simulink model "qless_forgetting_factor_16x16_nofifo"  (R2021a)
settings: Solver=FixedStepDiscrete  StartTime=0.0  StopTime=stoptime*inf  RelTol=1e-3
InitFcn:
  | qless_init_16chan_fi
undefined symbols (not defined in the file): fc, numArrayElements, physconst, srcAngles, Ts
libraries: hdlsllib x137, commfilt2 x4, commrfcorlib x3, commsync2 x3, commrflib2 x2, commrandsrc3 x2, simulink x2, phasedtxrxlib x2, commdigbbndcpm2 x1, embreciprocals x1, commdigbbndpm3 x1
(part 5 of 22)

== system qless_forgetting_factor_16x16_nofifo/MVDR_QLess_HDL/Complex Partial-Systolic Matrix Solve Using Q-less QR Decomposition with Forgetting Factor Manually Tiled n=16/Complex Partial-Systolic Q-less QR with Forgetting Factor/Complex Partial-Systolic Q-less QR with Forgetting Factor Manually tiled/Complex Partial-Systolic Q-less QR Decomposition with Forgetting Factor Section Constant pivot11/Partial-Systolic Q-less QR with Forgetting Factor Memory Controller ==
  xIn : Inport
  aIn : Inport  Port=2
  validIn : Inport  Port=3
  validElim : Inport  Port=4
  restart : Inport  Port=5
  Delay{,2..4,6} (5 alike) : Delay  DelayLength=1
  MATLAB Function : MATLAB Function  TreatAsAtomicUnit=on
  xOut : Outport  VectorParamsAs1DForOutWhenUnconnected=off
  yOut : Outport  Port=2  VectorParamsAs1DForOutWhenUnconnected=off
  process : Outport  Port=3  VectorParamsAs1DForOutWhenUnconnected=off
  validOut : Outport  Port=4  VectorParamsAs1DForOutWhenUnconnected=off
  ready : Outport  Port=5  VectorParamsAs1DForOutWhenUnconnected=off
  wires:
  Delay/1 -> MATLAB Function/1(xIn)
  Delay2/1 -> MATLAB Function/2(aIn)
  Delay3/1 -> MATLAB Function/3(validIn)
  Delay4/1 -> MATLAB Function/4(validRowRotationInput)
  Delay6/1 -> MATLAB Function/5(restart)
  xIn/1 -> Delay/1  "A"
  aIn/1 -> Delay2/1
  validIn/1 -> Delay3/1  "validIn"
  validElim/1 -> Delay4/1  "validElim"
  restart/1 -> Delay6/1  "validElim"
  MATLAB Function/1(xOut) -> xOut/1
  MATLAB Function/2(yOut) -> yOut/1
  MATLAB Function/3(processRowRotations) -> process/1
  MATLAB Function/4(validOut) -> validOut/1
  MATLAB Function/5(ready) -> ready/1

== system qless_forgetting_factor_16x16_nofifo/MVDR_QLess_HDL/Complex Partial-Systolic Matrix Solve Using Q-less QR Decomposition with Forgetting Factor Manually Tiled n=16/Complex Partial-Systolic Q-less QR with Forgetting Factor/Complex Partial-Systolic Q-less QR with Forgetting Factor Manually tiled/Complex Partial-Systolic Q-less QR Decomposition with Forgetting Factor Section Constant pivot11/Same Datatype ==
  Data : Inport
  Reference : Inport  Port=2
  Data Type Duplicate : DataTypeDuplicate
  DataOut : Outport  VectorParamsAs1DForOutWhenUnconnected=off
  wires:
  Reference/1 -> Data Type Duplicate/2
  Data/1 -> DataOut/1, Data Type Duplicate/1

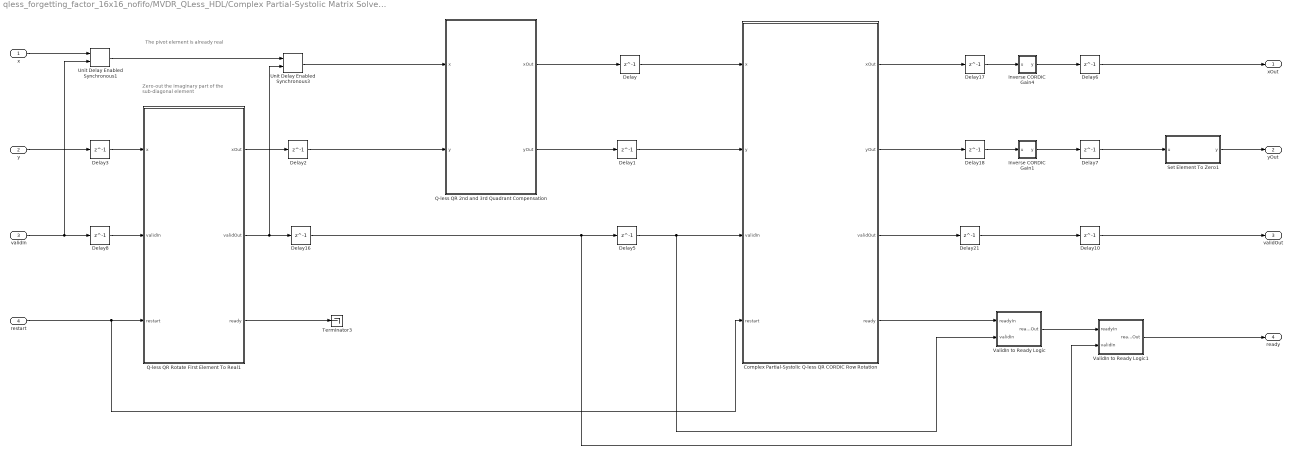
== system qless_forgetting_factor_16x16_nofifo/MVDR_QLess_HDL/Complex Partial-Systolic Matrix Solve Using Q-less QR Decomposition with Forgetting Factor Manually Tiled n=16/Complex Partial-Systolic Q-less QR with Forgetting Factor/Complex Partial-Systolic Q-less QR with Forgetting Factor Manually tiled/Complex Partial-Systolic Q-less QR Decomposition with Forgetting Factor Section Constant pivot12/Complex Partial-Systolic Q-less QR Row Rotations ==
  note: The pivot element is already real
  note: Zero-out the imaginary part
      | of the sub-diagonal element
  x : Inport
  y : Inport  Port=2
  validIn : Inport  Port=3
  restart : Inport  Port=4
  Complex Partial-Systolic Q-less QR CORDIC Row Rotation : Subsystem  TreatAsAtomicUnit=on  mask(Real Indexed CORDIC Row Rotation){n=n, pivot=pivot}
      mask prompts: n "fixed:emblib:ColumnsInA"
      mask help: fixed:emblib:RealIdxCORDIC
      mask DialogControl n Prompt: Number of columns in matrix A
  Delay{,1..3,5..8,10,16..18,21} (13 alike) : Delay  DelayLength=1
  Inverse CORDIC Gain1 : Subsystem  mask(Inverse CORDIC Gain){}
      mask help: fixed:emblib:InverseCORDICGainDescription
      mask Display: disp('1/An')
  Inverse CORDIC Gain4 : Subsystem  mask(Inverse CORDIC Gain){}
      mask help: fixed:emblib:InverseCORDICGainDescription
      mask Display: disp('1/An')
  Q-less QR 2nd and 3rd Quadrant Compensation : MATLAB Function  TreatAsAtomicUnit=on
  Q-less QR Rotate First Element To Real1 : Subsystem  TreatAsAtomicUnit=on  mask(Rotate First Element To Real){n=n, pivot=pivot}
      mask prompts: n "fixed:emblib:ColumnsInA"
      mask help: fixed:emblib:RotateFirstElementToRealDescription
      mask DialogControl n Prompt: Number of columns in matrix A
  Set Element To Zero1 : Subsystem  mask(Set Element To Zero){n=n, pivot=pivot}
      mask prompts: n "fixed:emblib:ColumnsInA"
      mask help: fixed:emblib:SetElementToZeroDescription
      mask DialogControl n Prompt: Number of columns in matrix A
  Terminator3 : Terminator
  Unit Delay Enabled Synchronous1 : hdlsllib/Discrete/Unit Delay Enabled Synchronous  InitialCondition=0.0  SampleTime=-1
      settings: SourceProductBaseCode=SL
  Unit Delay Enabled Synchronous3 : hdlsllib/Discrete/Unit Delay Enabled Synchronous  InitialCondition=0.0  SampleTime=-1
      settings: SourceProductBaseCode=SL
  ValidIn to Ready Logic : Subsystem
  ValidIn to Ready Logic1 : Subsystem
  xOut : Outport  VectorParamsAs1DForOutWhenUnconnected=off
  yOut : Outport  Port=2  VectorParamsAs1DForOutWhenUnconnected=off
  validOut : Outport  Port=3  VectorParamsAs1DForOutWhenUnconnected=off
  ready : Outport  Port=4  VectorParamsAs1DForOutWhenUnconnected=off
  wires:
  Delay6/1 -> xOut/1
  Complex Partial-Systolic Q-less QR CORDIC Row Rotation/1(xOut) -> Delay17/1
  Q-less QR 2nd and 3rd Quadrant Compensation/1(xOut) -> Delay/1
  Q-less QR 2nd and 3rd Quadrant Compensation/2(yOut) -> Delay1/1
  Delay/1 -> Complex Partial-Systolic Q-less QR CORDIC Row Rotation/1(x)
  Q-less QR Rotate First Element To Real1/2(validOut) -> Unit Delay Enabled Synchronous3/2, Delay16/1
  Q-less QR Rotate First Element To Real1/1(xOut) -> Delay2/1
  Delay1/1 -> Complex Partial-Systolic Q-less QR CORDIC Row Rotation/2(y)
  restart/1 -> Q-less QR Rotate First Element To Real1/3(restart), Complex Partial-Systolic Q-less QR CORDIC Row Rotation/4(restart)
  Delay5/1 -> ValidIn to Ready Logic/2(validIn), Complex Partial-Systolic Q-less QR CORDIC Row Rotation/3(validIn)
  Complex Partial-Systolic Q-less QR CORDIC Row Rotation/4(ready) -> ValidIn to Ready Logic/1(readyIn)
  Complex Partial-Systolic Q-less QR CORDIC Row Rotation/3(validOut) -> Delay21/1
  Complex Partial-Systolic Q-less QR CORDIC Row Rotation/2(yOut) -> Delay18/1
  y/1 -> Delay3/1
  Delay10/1 -> validOut/1
  ValidIn to Ready Logic/1(readyOut) -> ValidIn to Ready Logic1/1(readyIn)
  Delay7/1 -> Set Element To Zero1/1(u)
  Q-less QR Rotate First Element To Real1/3(ready) -> Terminator3/1
  ValidIn to Ready Logic1/1(readyOut) -> ready/1
  Delay21/1 -> Delay10/1
  Delay18/1 -> Inverse CORDIC Gain1/1(u)
  Delay17/1 -> Inverse CORDIC Gain4/1(u)
  Inverse CORDIC Gain4/1(y) -> Delay6/1
  Inverse CORDIC Gain1/1(y) -> Delay7/1
  validIn/1 -> Unit Delay Enabled Synchronous1/2, Delay8/1
  Delay16/1 -> ValidIn to Ready Logic1/2(validIn), Delay5/1
  Delay2/1 -> Q-less QR 2nd and 3rd Quadrant Compensation/2(y)
  Unit Delay Enabled Synchronous3/1 -> Q-less QR 2nd and 3rd Quadrant Compensation/1(x)
  Unit Delay Enabled Synchronous1/1 -> Unit Delay Enabled Synchronous3/1
  x/1 -> Unit Delay Enabled Synchronous1/1
  Delay3/1 -> Q-less QR Rotate First Element To Real1/1(x)
  Delay8/1 -> Q-less QR Rotate First Element To Real1/2(validIn)
  Set Element To Zero1/1(y) -> yOut/1

== system qless_forgetting_factor_16x16_nofifo/MVDR_QLess_HDL/Complex Partial-Systolic Matrix Solve Using Q-less QR Decomposition with Forgetting Factor Manually Tiled n=16/Complex Partial-Systolic Q-less QR with Forgetting Factor/Complex Partial-Systolic Q-less QR with Forgetting Factor Manually tiled/Complex Partial-Systolic Q-less QR Decomposition with Forgetting Factor Section Constant pivot12/Partial-Systolic Q-less QR with Forgetting Factor Memory Controller ==
  xIn : Inport
  aIn : Inport  Port=2
  validIn : Inport  Port=3
  validElim : Inport  Port=4
  restart : Inport  Port=5
  Delay{,2..4,6} (5 alike) : Delay  DelayLength=1
  MATLAB Function : MATLAB Function  TreatAsAtomicUnit=on
  xOut : Outport  VectorParamsAs1DForOutWhenUnconnected=off
  yOut : Outport  Port=2  VectorParamsAs1DForOutWhenUnconnected=off
  process : Outport  Port=3  VectorParamsAs1DForOutWhenUnconnected=off
  validOut : Outport  Port=4  VectorParamsAs1DForOutWhenUnconnected=off
  ready : Outport  Port=5  VectorParamsAs1DForOutWhenUnconnected=off
  wires:
  Delay/1 -> MATLAB Function/1(xIn)
  Delay2/1 -> MATLAB Function/2(aIn)
  Delay3/1 -> MATLAB Function/3(validIn)
  Delay4/1 -> MATLAB Function/4(validRowRotationInput)
  Delay6/1 -> MATLAB Function/5(restart)
  xIn/1 -> Delay/1  "A"
  aIn/1 -> Delay2/1
  validIn/1 -> Delay3/1  "validIn"
  validElim/1 -> Delay4/1  "validElim"
  restart/1 -> Delay6/1  "validElim"
  MATLAB Function/1(xOut) -> xOut/1
  MATLAB Function/2(yOut) -> yOut/1
  MATLAB Function/3(processRowRotations) -> process/1
  MATLAB Function/4(validOut) -> validOut/1
  MATLAB Function/5(ready) -> ready/1

== system qless_forgetting_factor_16x16_nofifo/MVDR_QLess_HDL/Complex Partial-Systolic Matrix Solve Using Q-less QR Decomposition with Forgetting Factor Manually Tiled n=16/Complex Partial-Systolic Q-less QR with Forgetting Factor/Complex Partial-Systolic Q-less QR with Forgetting Factor Manually tiled/Complex Partial-Systolic Q-less QR Decomposition with Forgetting Factor Section Constant pivot12/Same Datatype ==
  Data : Inport
  Reference : Inport  Port=2
  Data Type Duplicate : DataTypeDuplicate
  DataOut : Outport  VectorParamsAs1DForOutWhenUnconnected=off
  wires:
  Reference/1 -> Data Type Duplicate/2
  Data/1 -> DataOut/1, Data Type Duplicate/1

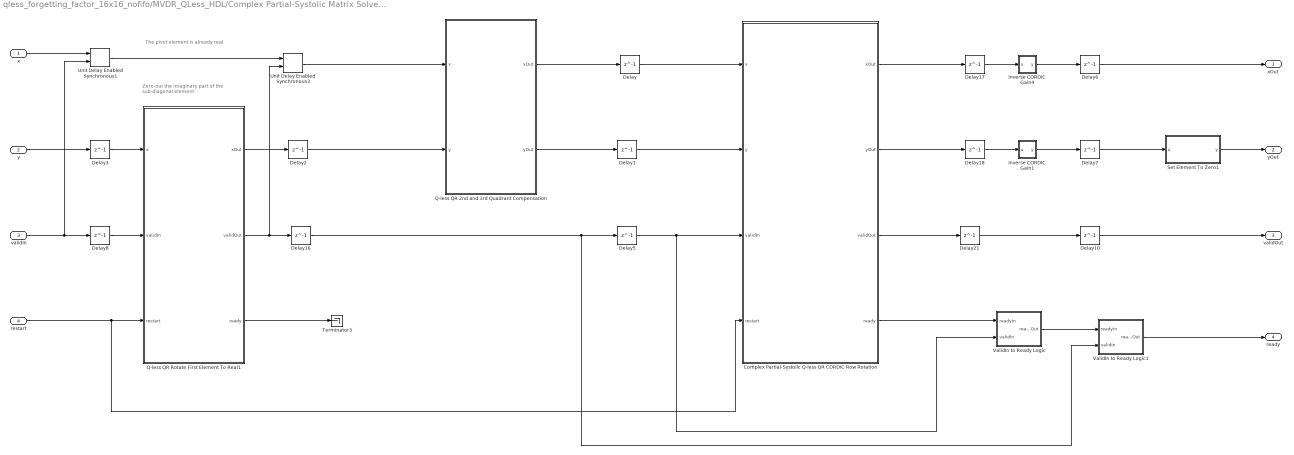
== system qless_forgetting_factor_16x16_nofifo/MVDR_QLess_HDL/Complex Partial-Systolic Matrix Solve Using Q-less QR Decomposition with Forgetting Factor Manually Tiled n=16/Complex Partial-Systolic Q-less QR with Forgetting Factor/Complex Partial-Systolic Q-less QR with Forgetting Factor Manually tiled/Complex Partial-Systolic Q-less QR Decomposition with Forgetting Factor Section Constant pivot13/Complex Partial-Systolic Q-less QR Row Rotations ==
  note: The pivot element is already real
  note: Zero-out the imaginary part
      | of the sub-diagonal element
  x : Inport
  y : Inport  Port=2
  validIn : Inport  Port=3
  restart : Inport  Port=4
  Complex Partial-Systolic Q-less QR CORDIC Row Rotation : Subsystem  TreatAsAtomicUnit=on  mask(Real Indexed CORDIC Row Rotation){n=n, pivot=pivot}
      mask prompts: n "fixed:emblib:ColumnsInA"
      mask help: fixed:emblib:RealIdxCORDIC
      mask DialogControl n Prompt: Number of columns in matrix A
  Delay{,1..3,5..8,10,16..18,21} (13 alike) : Delay  DelayLength=1
  Inverse CORDIC Gain1 : Subsystem  mask(Inverse CORDIC Gain){}
      mask help: fixed:emblib:InverseCORDICGainDescription
      mask Display: disp('1/An')
  Inverse CORDIC Gain4 : Subsystem  mask(Inverse CORDIC Gain){}
      mask help: fixed:emblib:InverseCORDICGainDescription
      mask Display: disp('1/An')
  Q-less QR 2nd and 3rd Quadrant Compensation : MATLAB Function  TreatAsAtomicUnit=on
  Q-less QR Rotate First Element To Real1 : Subsystem  TreatAsAtomicUnit=on  mask(Rotate First Element To Real){n=n, pivot=pivot}
      mask prompts: n "fixed:emblib:ColumnsInA"
      mask help: fixed:emblib:RotateFirstElementToRealDescription
      mask DialogControl n Prompt: Number of columns in matrix A
  Set Element To Zero1 : Subsystem  mask(Set Element To Zero){n=n, pivot=pivot}
      mask prompts: n "fixed:emblib:ColumnsInA"
      mask help: fixed:emblib:SetElementToZeroDescription
      mask DialogControl n Prompt: Number of columns in matrix A
  Terminator3 : Terminator
  Unit Delay Enabled Synchronous1 : hdlsllib/Discrete/Unit Delay Enabled Synchronous  InitialCondition=0.0  SampleTime=-1
      settings: SourceProductBaseCode=SL
  Unit Delay Enabled Synchronous3 : hdlsllib/Discrete/Unit Delay Enabled Synchronous  InitialCondition=0.0  SampleTime=-1
      settings: SourceProductBaseCode=SL
  ValidIn to Ready Logic : Subsystem
  ValidIn to Ready Logic1 : Subsystem
  xOut : Outport  VectorParamsAs1DForOutWhenUnconnected=off
  yOut : Outport  Port=2  VectorParamsAs1DForOutWhenUnconnected=off
  validOut : Outport  Port=3  VectorParamsAs1DForOutWhenUnconnected=off
  ready : Outport  Port=4  VectorParamsAs1DForOutWhenUnconnected=off
  wires:
  Delay6/1 -> xOut/1
  Complex Partial-Systolic Q-less QR CORDIC Row Rotation/1(xOut) -> Delay17/1
  Q-less QR 2nd and 3rd Quadrant Compensation/1(xOut) -> Delay/1
  Q-less QR 2nd and 3rd Quadrant Compensation/2(yOut) -> Delay1/1
  Delay/1 -> Complex Partial-Systolic Q-less QR CORDIC Row Rotation/1(x)
  Q-less QR Rotate First Element To Real1/2(validOut) -> Unit Delay Enabled Synchronous3/2, Delay16/1
  Q-less QR Rotate First Element To Real1/1(xOut) -> Delay2/1
  Delay1/1 -> Complex Partial-Systolic Q-less QR CORDIC Row Rotation/2(y)
  restart/1 -> Q-less QR Rotate First Element To Real1/3(restart), Complex Partial-Systolic Q-less QR CORDIC Row Rotation/4(restart)
  Delay5/1 -> ValidIn to Ready Logic/2(validIn), Complex Partial-Systolic Q-less QR CORDIC Row Rotation/3(validIn)
  Complex Partial-Systolic Q-less QR CORDIC Row Rotation/4(ready) -> ValidIn to Ready Logic/1(readyIn)
  Complex Partial-Systolic Q-less QR CORDIC Row Rotation/3(validOut) -> Delay21/1
  Complex Partial-Systolic Q-less QR CORDIC Row Rotation/2(yOut) -> Delay18/1
  y/1 -> Delay3/1
  Delay10/1 -> validOut/1
  ValidIn to Ready Logic/1(readyOut) -> ValidIn to Ready Logic1/1(readyIn)
  Delay7/1 -> Set Element To Zero1/1(u)
  Q-less QR Rotate First Element To Real1/3(ready) -> Terminator3/1
  ValidIn to Ready Logic1/1(readyOut) -> ready/1
  Delay21/1 -> Delay10/1
  Delay18/1 -> Inverse CORDIC Gain1/1(u)
  Delay17/1 -> Inverse CORDIC Gain4/1(u)
  Inverse CORDIC Gain4/1(y) -> Delay6/1
  Inverse CORDIC Gain1/1(y) -> Delay7/1
  validIn/1 -> Unit Delay Enabled Synchronous1/2, Delay8/1
  Delay16/1 -> ValidIn to Ready Logic1/2(validIn), Delay5/1
  Delay2/1 -> Q-less QR 2nd and 3rd Quadrant Compensation/2(y)
  Unit Delay Enabled Synchronous3/1 -> Q-less QR 2nd and 3rd Quadrant Compensation/1(x)
  Unit Delay Enabled Synchronous1/1 -> Unit Delay Enabled Synchronous3/1
  x/1 -> Unit Delay Enabled Synchronous1/1
  Delay3/1 -> Q-less QR Rotate First Element To Real1/1(x)
  Delay8/1 -> Q-less QR Rotate First Element To Real1/2(validIn)
  Set Element To Zero1/1(y) -> yOut/1

== system qless_forgetting_factor_16x16_nofifo/MVDR_QLess_HDL/Complex Partial-Systolic Matrix Solve Using Q-less QR Decomposition with Forgetting Factor Manually Tiled n=16/Complex Partial-Systolic Q-less QR with Forgetting Factor/Complex Partial-Systolic Q-less QR with Forgetting Factor Manually tiled/Complex Partial-Systolic Q-less QR Decomposition with Forgetting Factor Section Constant pivot13/Partial-Systolic Q-less QR with Forgetting Factor Memory Controller ==
  xIn : Inport
  aIn : Inport  Port=2
  validIn : Inport  Port=3
  validElim : Inport  Port=4
  restart : Inport  Port=5
  Delay{,2..4,6} (5 alike) : Delay  DelayLength=1
  MATLAB Function : MATLAB Function  TreatAsAtomicUnit=on
  xOut : Outport  VectorParamsAs1DForOutWhenUnconnected=off
  yOut : Outport  Port=2  VectorParamsAs1DForOutWhenUnconnected=off
  process : Outport  Port=3  VectorParamsAs1DForOutWhenUnconnected=off
  validOut : Outport  Port=4  VectorParamsAs1DForOutWhenUnconnected=off
  ready : Outport  Port=5  VectorParamsAs1DForOutWhenUnconnected=off
  wires:
  Delay/1 -> MATLAB Function/1(xIn)
  Delay2/1 -> MATLAB Function/2(aIn)
  Delay3/1 -> MATLAB Function/3(validIn)
  Delay4/1 -> MATLAB Function/4(validRowRotationInput)
  Delay6/1 -> MATLAB Function/5(restart)
  xIn/1 -> Delay/1  "A"
  aIn/1 -> Delay2/1
  validIn/1 -> Delay3/1  "validIn"
  validElim/1 -> Delay4/1  "validElim"
  restart/1 -> Delay6/1  "validElim"
  MATLAB Function/1(xOut) -> xOut/1
  MATLAB Function/2(yOut) -> yOut/1
  MATLAB Function/3(processRowRotations) -> process/1
  MATLAB Function/4(validOut) -> validOut/1
  MATLAB Function/5(ready) -> ready/1

== system qless_forgetting_factor_16x16_nofifo/MVDR_QLess_HDL/Complex Partial-Systolic Matrix Solve Using Q-less QR Decomposition with Forgetting Factor Manually Tiled n=16/Complex Partial-Systolic Q-less QR with Forgetting Factor/Complex Partial-Systolic Q-less QR with Forgetting Factor Manually tiled/Complex Partial-Systolic Q-less QR Decomposition with Forgetting Factor Section Constant pivot13/Same Datatype ==
  Data : Inport
  Reference : Inport  Port=2
  Data Type Duplicate : DataTypeDuplicate
  DataOut : Outport  VectorParamsAs1DForOutWhenUnconnected=off
  wires:
  Reference/1 -> Data Type Duplicate/2
  Data/1 -> DataOut/1, Data Type Duplicate/1

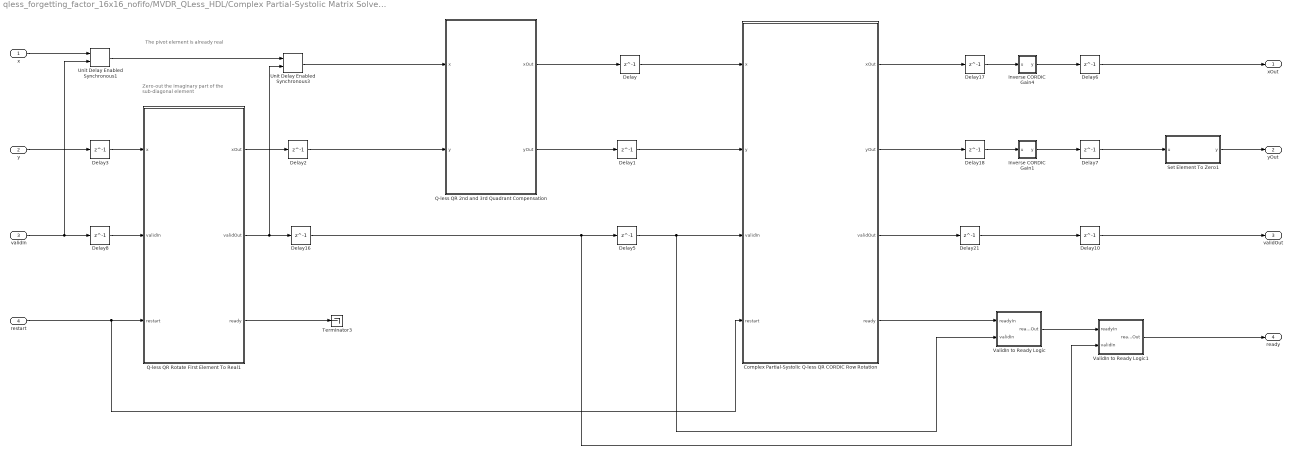
== system qless_forgetting_factor_16x16_nofifo/MVDR_QLess_HDL/Complex Partial-Systolic Matrix Solve Using Q-less QR Decomposition with Forgetting Factor Manually Tiled n=16/Complex Partial-Systolic Q-less QR with Forgetting Factor/Complex Partial-Systolic Q-less QR with Forgetting Factor Manually tiled/Complex Partial-Systolic Q-less QR Decomposition with Forgetting Factor Section Constant pivot14/Complex Partial-Systolic Q-less QR Row Rotations ==
  note: The pivot element is already real
  note: Zero-out the imaginary part
      | of the sub-diagonal element
  x : Inport
  y : Inport  Port=2
  validIn : Inport  Port=3
  restart : Inport  Port=4
  Complex Partial-Systolic Q-less QR CORDIC Row Rotation : Subsystem  TreatAsAtomicUnit=on  mask(Real Indexed CORDIC Row Rotation){n=n, pivot=pivot}
      mask prompts: n "fixed:emblib:ColumnsInA"
      mask help: fixed:emblib:RealIdxCORDIC
      mask DialogControl n Prompt: Number of columns in matrix A
  Delay{,1..3,5..8,10,16..18,21} (13 alike) : Delay  DelayLength=1
  Inverse CORDIC Gain1 : Subsystem  mask(Inverse CORDIC Gain){}
      mask help: fixed:emblib:InverseCORDICGainDescription
      mask Display: disp('1/An')
  Inverse CORDIC Gain4 : Subsystem  mask(Inverse CORDIC Gain){}
      mask help: fixed:emblib:InverseCORDICGainDescription
      mask Display: disp('1/An')
  Q-less QR 2nd and 3rd Quadrant Compensation : MATLAB Function  TreatAsAtomicUnit=on
  Q-less QR Rotate First Element To Real1 : Subsystem  TreatAsAtomicUnit=on  mask(Rotate First Element To Real){n=n, pivot=pivot}
      mask prompts: n "fixed:emblib:ColumnsInA"
      mask help: fixed:emblib:RotateFirstElementToRealDescription
      mask DialogControl n Prompt: Number of columns in matrix A
  Set Element To Zero1 : Subsystem  mask(Set Element To Zero){n=n, pivot=pivot}
      mask prompts: n "fixed:emblib:ColumnsInA"
      mask help: fixed:emblib:SetElementToZeroDescription
      mask DialogControl n Prompt: Number of columns in matrix A
  Terminator3 : Terminator
  Unit Delay Enabled Synchronous1 : hdlsllib/Discrete/Unit Delay Enabled Synchronous  InitialCondition=0.0  SampleTime=-1
      settings: SourceProductBaseCode=SL
  Unit Delay Enabled Synchronous3 : hdlsllib/Discrete/Unit Delay Enabled Synchronous  InitialCondition=0.0  SampleTime=-1
      settings: SourceProductBaseCode=SL
  ValidIn to Ready Logic : Subsystem
  ValidIn to Ready Logic1 : Subsystem
  xOut : Outport  VectorParamsAs1DForOutWhenUnconnected=off
  yOut : Outport  Port=2  VectorParamsAs1DForOutWhenUnconnected=off
  validOut : Outport  Port=3  VectorParamsAs1DForOutWhenUnconnected=off
  ready : Outport  Port=4  VectorParamsAs1DForOutWhenUnconnected=off
  wires:
  Delay6/1 -> xOut/1
  Complex Partial-Systolic Q-less QR CORDIC Row Rotation/1(xOut) -> Delay17/1
  Q-less QR 2nd and 3rd Quadrant Compensation/1(xOut) -> Delay/1
  Q-less QR 2nd and 3rd Quadrant Compensation/2(yOut) -> Delay1/1
  Delay/1 -> Complex Partial-Systolic Q-less QR CORDIC Row Rotation/1(x)
  Q-less QR Rotate First Element To Real1/2(validOut) -> Unit Delay Enabled Synchronous3/2, Delay16/1
  Q-less QR Rotate First Element To Real1/1(xOut) -> Delay2/1
  Delay1/1 -> Complex Partial-Systolic Q-less QR CORDIC Row Rotation/2(y)
  restart/1 -> Q-less QR Rotate First Element To Real1/3(restart), Complex Partial-Systolic Q-less QR CORDIC Row Rotation/4(restart)
  Delay5/1 -> ValidIn to Ready Logic/2(validIn), Complex Partial-Systolic Q-less QR CORDIC Row Rotation/3(validIn)
  Complex Partial-Systolic Q-less QR CORDIC Row Rotation/4(ready) -> ValidIn to Ready Logic/1(readyIn)
  Complex Partial-Systolic Q-less QR CORDIC Row Rotation/3(validOut) -> Delay21/1
  Complex Partial-Systolic Q-less QR CORDIC Row Rotation/2(yOut) -> Delay18/1
  y/1 -> Delay3/1
  Delay10/1 -> validOut/1
  ValidIn to Ready Logic/1(readyOut) -> ValidIn to Ready Logic1/1(readyIn)
  Delay7/1 -> Set Element To Zero1/1(u)
  Q-less QR Rotate First Element To Real1/3(ready) -> Terminator3/1
  ValidIn to Ready Logic1/1(readyOut) -> ready/1
  Delay21/1 -> Delay10/1
  Delay18/1 -> Inverse CORDIC Gain1/1(u)
  Delay17/1 -> Inverse CORDIC Gain4/1(u)
  Inverse CORDIC Gain4/1(y) -> Delay6/1
  Inverse CORDIC Gain1/1(y) -> Delay7/1
  validIn/1 -> Unit Delay Enabled Synchronous1/2, Delay8/1
  Delay16/1 -> ValidIn to Ready Logic1/2(validIn), Delay5/1
  Delay2/1 -> Q-less QR 2nd and 3rd Quadrant Compensation/2(y)
  Unit Delay Enabled Synchronous3/1 -> Q-less QR 2nd and 3rd Quadrant Compensation/1(x)
  Unit Delay Enabled Synchronous1/1 -> Unit Delay Enabled Synchronous3/1
  x/1 -> Unit Delay Enabled Synchronous1/1
  Delay3/1 -> Q-less QR Rotate First Element To Real1/1(x)
  Delay8/1 -> Q-less QR Rotate First Element To Real1/2(validIn)
  Set Element To Zero1/1(y) -> yOut/1

== system qless_forgetting_factor_16x16_nofifo/MVDR_QLess_HDL/Complex Partial-Systolic Matrix Solve Using Q-less QR Decomposition with Forgetting Factor Manually Tiled n=16/Complex Partial-Systolic Q-less QR with Forgetting Factor/Complex Partial-Systolic Q-less QR with Forgetting Factor Manually tiled/Complex Partial-Systolic Q-less QR Decomposition with Forgetting Factor Section Constant pivot14/Partial-Systolic Q-less QR with Forgetting Factor Memory Controller ==
  xIn : Inport
  aIn : Inport  Port=2
  validIn : Inport  Port=3
  validElim : Inport  Port=4
  restart : Inport  Port=5
  Delay{,2..4,6} (5 alike) : Delay  DelayLength=1
  MATLAB Function : MATLAB Function  TreatAsAtomicUnit=on
  xOut : Outport  VectorParamsAs1DForOutWhenUnconnected=off
  yOut : Outport  Port=2  VectorParamsAs1DForOutWhenUnconnected=off
  process : Outport  Port=3  VectorParamsAs1DForOutWhenUnconnected=off
  validOut : Outport  Port=4  VectorParamsAs1DForOutWhenUnconnected=off
  ready : Outport  Port=5  VectorParamsAs1DForOutWhenUnconnected=off
  wires:
  Delay/1 -> MATLAB Function/1(xIn)
  Delay2/1 -> MATLAB Function/2(aIn)
  Delay3/1 -> MATLAB Function/3(validIn)
  Delay4/1 -> MATLAB Function/4(validRowRotationInput)
  Delay6/1 -> MATLAB Function/5(restart)
  xIn/1 -> Delay/1  "A"
  aIn/1 -> Delay2/1
  validIn/1 -> Delay3/1  "validIn"
  validElim/1 -> Delay4/1  "validElim"
  restart/1 -> Delay6/1  "validElim"
  MATLAB Function/1(xOut) -> xOut/1
  MATLAB Function/2(yOut) -> yOut/1
  MATLAB Function/3(processRowRotations) -> process/1
  MATLAB Function/4(validOut) -> validOut/1
  MATLAB Function/5(ready) -> ready/1

== system qless_forgetting_factor_16x16_nofifo/MVDR_QLess_HDL/Complex Partial-Systolic Matrix Solve Using Q-less QR Decomposition with Forgetting Factor Manually Tiled n=16/Complex Partial-Systolic Q-less QR with Forgetting Factor/Complex Partial-Systolic Q-less QR with Forgetting Factor Manually tiled/Complex Partial-Systolic Q-less QR Decomposition with Forgetting Factor Section Constant pivot14/Same Datatype ==
  Data : Inport
  Reference : Inport  Port=2
  Data Type Duplicate : DataTypeDuplicate
  DataOut : Outport  VectorParamsAs1DForOutWhenUnconnected=off
  wires:
  Reference/1 -> Data Type Duplicate/2
  Data/1 -> DataOut/1, Data Type Duplicate/1

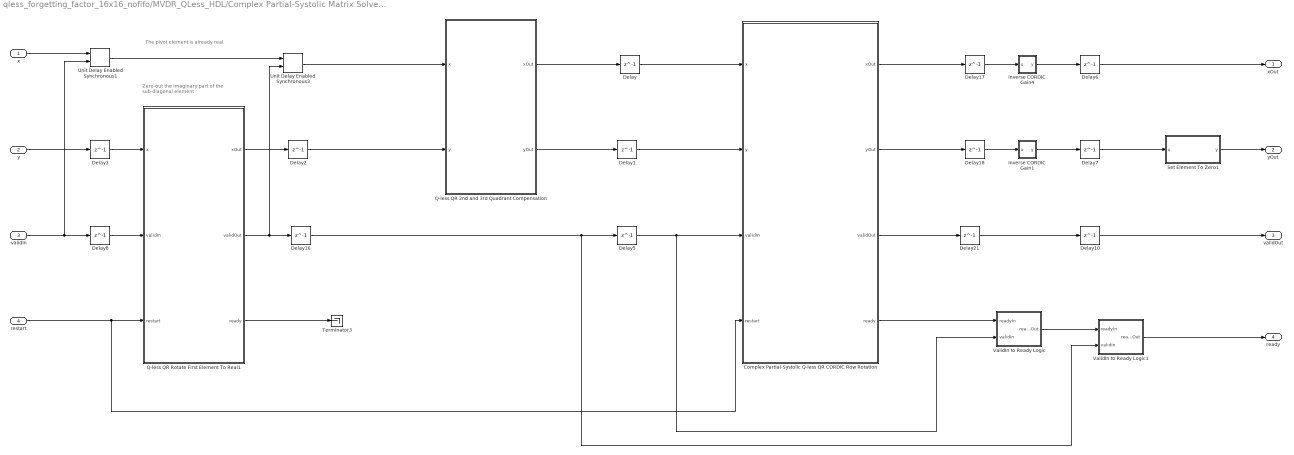
== system qless_forgetting_factor_16x16_nofifo/MVDR_QLess_HDL/Complex Partial-Systolic Matrix Solve Using Q-less QR Decomposition with Forgetting Factor Manually Tiled n=16/Complex Partial-Systolic Q-less QR with Forgetting Factor/Complex Partial-Systolic Q-less QR with Forgetting Factor Manually tiled/Complex Partial-Systolic Q-less QR Decomposition with Forgetting Factor Section Constant pivot15/Complex Partial-Systolic Q-less QR Row Rotations ==
  note: The pivot element is already real
  note: Zero-out the imaginary part
      | of the sub-diagonal element
  x : Inport
  y : Inport  Port=2
  validIn : Inport  Port=3
  restart : Inport  Port=4
  Complex Partial-Systolic Q-less QR CORDIC Row Rotation : Subsystem  TreatAsAtomicUnit=on  mask(Real Indexed CORDIC Row Rotation){n=n, pivot=pivot}
      mask prompts: n "fixed:emblib:ColumnsInA"
      mask help: fixed:emblib:RealIdxCORDIC
      mask DialogControl n Prompt: Number of columns in matrix A
  Delay{,1..3,5..8,10,16..18,21} (13 alike) : Delay  DelayLength=1
  Inverse CORDIC Gain1 : Subsystem  mask(Inverse CORDIC Gain){}
      mask help: fixed:emblib:InverseCORDICGainDescription
      mask Display: disp('1/An')
  Inverse CORDIC Gain4 : Subsystem  mask(Inverse CORDIC Gain){}
      mask help: fixed:emblib:InverseCORDICGainDescription
      mask Display: disp('1/An')
  Q-less QR 2nd and 3rd Quadrant Compensation : MATLAB Function  TreatAsAtomicUnit=on
  Q-less QR Rotate First Element To Real1 : Subsystem  TreatAsAtomicUnit=on  mask(Rotate First Element To Real){n=n, pivot=pivot}
      mask prompts: n "fixed:emblib:ColumnsInA"
      mask help: fixed:emblib:RotateFirstElementToRealDescription
      mask DialogControl n Prompt: Number of columns in matrix A
  Set Element To Zero1 : Subsystem  mask(Set Element To Zero){n=n, pivot=pivot}
      mask prompts: n "fixed:emblib:ColumnsInA"
      mask help: fixed:emblib:SetElementToZeroDescription
      mask DialogControl n Prompt: Number of columns in matrix A
  Terminator3 : Terminator
  Unit Delay Enabled Synchronous1 : hdlsllib/Discrete/Unit Delay Enabled Synchronous  InitialCondition=0.0  SampleTime=-1
      settings: SourceProductBaseCode=SL
  Unit Delay Enabled Synchronous3 : hdlsllib/Discrete/Unit Delay Enabled Synchronous  InitialCondition=0.0  SampleTime=-1
      settings: SourceProductBaseCode=SL
  ValidIn to Ready Logic : Subsystem
  ValidIn to Ready Logic1 : Subsystem
  xOut : Outport  VectorParamsAs1DForOutWhenUnconnected=off
  yOut : Outport  Port=2  VectorParamsAs1DForOutWhenUnconnected=off
  validOut : Outport  Port=3  VectorParamsAs1DForOutWhenUnconnected=off
  ready : Outport  Port=4  VectorParamsAs1DForOutWhenUnconnected=off
  wires:
  Delay6/1 -> xOut/1
  Complex Partial-Systolic Q-less QR CORDIC Row Rotation/1(xOut) -> Delay17/1
  Q-less QR 2nd and 3rd Quadrant Compensation/1(xOut) -> Delay/1
  Q-less QR 2nd and 3rd Quadrant Compensation/2(yOut) -> Delay1/1
  Delay/1 -> Complex Partial-Systolic Q-less QR CORDIC Row Rotation/1(x)
  Q-less QR Rotate First Element To Real1/2(validOut) -> Unit Delay Enabled Synchronous3/2, Delay16/1
  Q-less QR Rotate First Element To Real1/1(xOut) -> Delay2/1
  Delay1/1 -> Complex Partial-Systolic Q-less QR CORDIC Row Rotation/2(y)
  restart/1 -> Q-less QR Rotate First Element To Real1/3(restart), Complex Partial-Systolic Q-less QR CORDIC Row Rotation/4(restart)
  Delay5/1 -> ValidIn to Ready Logic/2(validIn), Complex Partial-Systolic Q-less QR CORDIC Row Rotation/3(validIn)
  Complex Partial-Systolic Q-less QR CORDIC Row Rotation/4(ready) -> ValidIn to Ready Logic/1(readyIn)
  Complex Partial-Systolic Q-less QR CORDIC Row Rotation/3(validOut) -> Delay21/1
  Complex Partial-Systolic Q-less QR CORDIC Row Rotation/2(yOut) -> Delay18/1
  y/1 -> Delay3/1
  Delay10/1 -> validOut/1
  ValidIn to Ready Logic/1(readyOut) -> ValidIn to Ready Logic1/1(readyIn)
  Delay7/1 -> Set Element To Zero1/1(u)
  Q-less QR Rotate First Element To Real1/3(ready) -> Terminator3/1
  ValidIn to Ready Logic1/1(readyOut) -> ready/1
  Delay21/1 -> Delay10/1
  Delay18/1 -> Inverse CORDIC Gain1/1(u)
  Delay17/1 -> Inverse CORDIC Gain4/1(u)
  Inverse CORDIC Gain4/1(y) -> Delay6/1
  Inverse CORDIC Gain1/1(y) -> Delay7/1
  validIn/1 -> Unit Delay Enabled Synchronous1/2, Delay8/1
  Delay16/1 -> ValidIn to Ready Logic1/2(validIn), Delay5/1
  Delay2/1 -> Q-less QR 2nd and 3rd Quadrant Compensation/2(y)
  Unit Delay Enabled Synchronous3/1 -> Q-less QR 2nd and 3rd Quadrant Compensation/1(x)
  Unit Delay Enabled Synchronous1/1 -> Unit Delay Enabled Synchronous3/1
  x/1 -> Unit Delay Enabled Synchronous1/1
  Delay3/1 -> Q-less QR Rotate First Element To Real1/1(x)
  Delay8/1 -> Q-less QR Rotate First Element To Real1/2(validIn)
  Set Element To Zero1/1(y) -> yOut/1

== system qless_forgetting_factor_16x16_nofifo/MVDR_QLess_HDL/Complex Partial-Systolic Matrix Solve Using Q-less QR Decomposition with Forgetting Factor Manually Tiled n=16/Complex Partial-Systolic Q-less QR with Forgetting Factor/Complex Partial-Systolic Q-less QR with Forgetting Factor Manually tiled/Complex Partial-Systolic Q-less QR Decomposition with Forgetting Factor Section Constant pivot15/Partial-Systolic Q-less QR with Forgetting Factor Memory Controller ==
  xIn : Inport
  aIn : Inport  Port=2
  validIn : Inport  Port=3
  validElim : Inport  Port=4
  restart : Inport  Port=5
  Delay{,2..4,6} (5 alike) : Delay  DelayLength=1
  MATLAB Function : MATLAB Function  TreatAsAtomicUnit=on
  xOut : Outport  VectorParamsAs1DForOutWhenUnconnected=off
  yOut : Outport  Port=2  VectorParamsAs1DForOutWhenUnconnected=off
  process : Outport  Port=3  VectorParamsAs1DForOutWhenUnconnected=off
  validOut : Outport  Port=4  VectorParamsAs1DForOutWhenUnconnected=off
  ready : Outport  Port=5  VectorParamsAs1DForOutWhenUnconnected=off
  wires:
  Delay/1 -> MATLAB Function/1(xIn)
  Delay2/1 -> MATLAB Function/2(aIn)
  Delay3/1 -> MATLAB Function/3(validIn)
  Delay4/1 -> MATLAB Function/4(validRowRotationInput)
  Delay6/1 -> MATLAB Function/5(restart)
  xIn/1 -> Delay/1  "A"
  aIn/1 -> Delay2/1
  validIn/1 -> Delay3/1  "validIn"
  validElim/1 -> Delay4/1  "validElim"
  restart/1 -> Delay6/1  "validElim"
  MATLAB Function/1(xOut) -> xOut/1
  MATLAB Function/2(yOut) -> yOut/1
  MATLAB Function/3(processRowRotations) -> process/1
  MATLAB Function/4(validOut) -> validOut/1
  MATLAB Function/5(ready) -> ready/1

== system qless_forgetting_factor_16x16_nofifo/MVDR_QLess_HDL/Complex Partial-Systolic Matrix Solve Using Q-less QR Decomposition with Forgetting Factor Manually Tiled n=16/Complex Partial-Systolic Q-less QR with Forgetting Factor/Complex Partial-Systolic Q-less QR with Forgetting Factor Manually tiled/Complex Partial-Systolic Q-less QR Decomposition with Forgetting Factor Section Constant pivot15/Same Datatype ==
  Data : Inport
  Reference : Inport  Port=2
  Data Type Duplicate : DataTypeDuplicate
  DataOut : Outport  VectorParamsAs1DForOutWhenUnconnected=off
  wires:
  Reference/1 -> Data Type Duplicate/2
  Data/1 -> DataOut/1, Data Type Duplicate/1

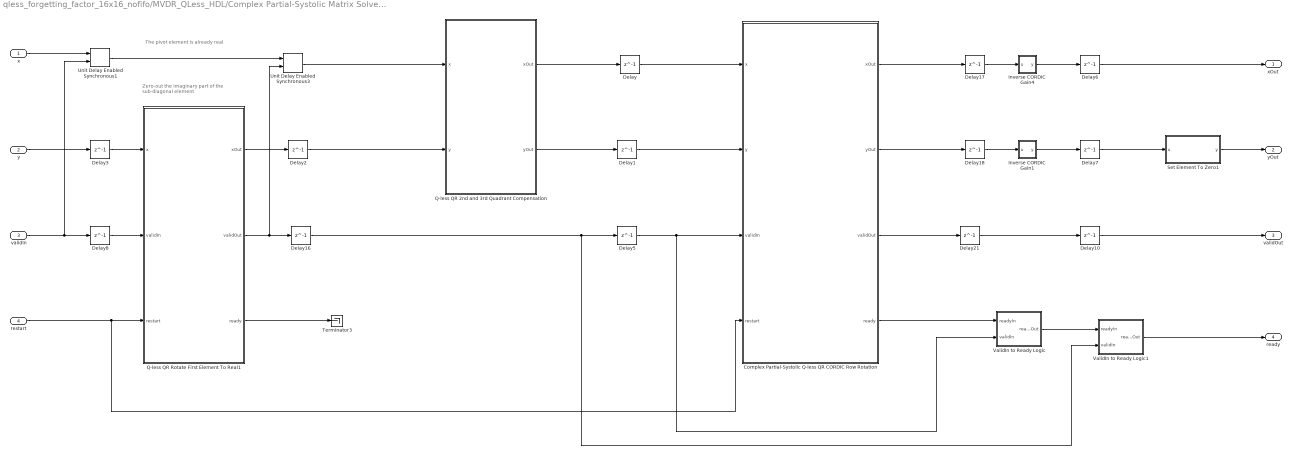
== system qless_forgetting_factor_16x16_nofifo/MVDR_QLess_HDL/Complex Partial-Systolic Matrix Solve Using Q-less QR Decomposition with Forgetting Factor Manually Tiled n=16/Complex Partial-Systolic Q-less QR with Forgetting Factor/Complex Partial-Systolic Q-less QR with Forgetting Factor Manually tiled/Complex Partial-Systolic Q-less QR Decomposition with Forgetting Factor Section Constant pivot16/Complex Partial-Systolic Q-less QR Row Rotations ==
  note: The pivot element is already real
  note: Zero-out the imaginary part
      | of the sub-diagonal element
  x : Inport
  y : Inport  Port=2
  validIn : Inport  Port=3
  restart : Inport  Port=4
  Complex Partial-Systolic Q-less QR CORDIC Row Rotation : Subsystem  TreatAsAtomicUnit=on  mask(Real Indexed CORDIC Row Rotation){n=n, pivot=pivot}
      mask prompts: n "fixed:emblib:ColumnsInA"
      mask help: fixed:emblib:RealIdxCORDIC
      mask DialogControl n Prompt: Number of columns in matrix A
  Delay{,1..3,5..8,10,16..18,21} (13 alike) : Delay  DelayLength=1
  Inverse CORDIC Gain1 : Subsystem  mask(Inverse CORDIC Gain){}
      mask help: fixed:emblib:InverseCORDICGainDescription
      mask Display: disp('1/An')
  Inverse CORDIC Gain4 : Subsystem  mask(Inverse CORDIC Gain){}
      mask help: fixed:emblib:InverseCORDICGainDescription
      mask Display: disp('1/An')
  Q-less QR 2nd and 3rd Quadrant Compensation : MATLAB Function  TreatAsAtomicUnit=on
  Q-less QR Rotate First Element To Real1 : Subsystem  TreatAsAtomicUnit=on  mask(Rotate First Element To Real){n=n, pivot=pivot}
      mask prompts: n "fixed:emblib:ColumnsInA"
      mask help: fixed:emblib:RotateFirstElementToRealDescription
      mask DialogControl n Prompt: Number of columns in matrix A
  Set Element To Zero1 : Subsystem  mask(Set Element To Zero){n=n, pivot=pivot}
      mask prompts: n "fixed:emblib:ColumnsInA"
      mask help: fixed:emblib:SetElementToZeroDescription
      mask DialogControl n Prompt: Number of columns in matrix A
  Terminator3 : Terminator
  Unit Delay Enabled Synchronous1 : hdlsllib/Discrete/Unit Delay Enabled Synchronous  InitialCondition=0.0  SampleTime=-1
      settings: SourceProductBaseCode=SL
  Unit Delay Enabled Synchronous3 : hdlsllib/Discrete/Unit Delay Enabled Synchronous  InitialCondition=0.0  SampleTime=-1
      settings: SourceProductBaseCode=SL
  ValidIn to Ready Logic : Subsystem
  ValidIn to Ready Logic1 : Subsystem
  xOut : Outport  VectorParamsAs1DForOutWhenUnconnected=off
  yOut : Outport  Port=2  VectorParamsAs1DForOutWhenUnconnected=off
  validOut : Outport  Port=3  VectorParamsAs1DForOutWhenUnconnected=off
  ready : Outport  Port=4  VectorParamsAs1DForOutWhenUnconnected=off
  wires:
  Delay6/1 -> xOut/1
  Complex Partial-Systolic Q-less QR CORDIC Row Rotation/1(xOut) -> Delay17/1
  Q-less QR 2nd and 3rd Quadrant Compensation/1(xOut) -> Delay/1
  Q-less QR 2nd and 3rd Quadrant Compensation/2(yOut) -> Delay1/1
  Delay/1 -> Complex Partial-Systolic Q-less QR CORDIC Row Rotation/1(x)
  Q-less QR Rotate First Element To Real1/2(validOut) -> Unit Delay Enabled Synchronous3/2, Delay16/1
  Q-less QR Rotate First Element To Real1/1(xOut) -> Delay2/1
  Delay1/1 -> Complex Partial-Systolic Q-less QR CORDIC Row Rotation/2(y)
  restart/1 -> Q-less QR Rotate First Element To Real1/3(restart), Complex Partial-Systolic Q-less QR CORDIC Row Rotation/4(restart)
  Delay5/1 -> ValidIn to Ready Logic/2(validIn), Complex Partial-Systolic Q-less QR CORDIC Row Rotation/3(validIn)
  Complex Partial-Systolic Q-less QR CORDIC Row Rotation/4(ready) -> ValidIn to Ready Logic/1(readyIn)
  Complex Partial-Systolic Q-less QR CORDIC Row Rotation/3(validOut) -> Delay21/1
  Complex Partial-Systolic Q-less QR CORDIC Row Rotation/2(yOut) -> Delay18/1
  y/1 -> Delay3/1
  Delay10/1 -> validOut/1
  ValidIn to Ready Logic/1(readyOut) -> ValidIn to Ready Logic1/1(readyIn)
  Delay7/1 -> Set Element To Zero1/1(u)
  Q-less QR Rotate First Element To Real1/3(ready) -> Terminator3/1
  ValidIn to Ready Logic1/1(readyOut) -> ready/1
  Delay21/1 -> Delay10/1
  Delay18/1 -> Inverse CORDIC Gain1/1(u)
  Delay17/1 -> Inverse CORDIC Gain4/1(u)
  Inverse CORDIC Gain4/1(y) -> Delay6/1
  Inverse CORDIC Gain1/1(y) -> Delay7/1
  validIn/1 -> Unit Delay Enabled Synchronous1/2, Delay8/1
  Delay16/1 -> ValidIn to Ready Logic1/2(validIn), Delay5/1
  Delay2/1 -> Q-less QR 2nd and 3rd Quadrant Compensation/2(y)
  Unit Delay Enabled Synchronous3/1 -> Q-less QR 2nd and 3rd Quadrant Compensation/1(x)
  Unit Delay Enabled Synchronous1/1 -> Unit Delay Enabled Synchronous3/1
  x/1 -> Unit Delay Enabled Synchronous1/1
  Delay3/1 -> Q-less QR Rotate First Element To Real1/1(x)
  Delay8/1 -> Q-less QR Rotate First Element To Real1/2(validIn)
  Set Element To Zero1/1(y) -> yOut/1

== system qless_forgetting_factor_16x16_nofifo/MVDR_QLess_HDL/Complex Partial-Systolic Matrix Solve Using Q-less QR Decomposition with Forgetting Factor Manually Tiled n=16/Complex Partial-Systolic Q-less QR with Forgetting Factor/Complex Partial-Systolic Q-less QR with Forgetting Factor Manually tiled/Complex Partial-Systolic Q-less QR Decomposition with Forgetting Factor Section Constant pivot16/Partial-Systolic Q-less QR with Forgetting Factor Memory Controller ==
  xIn : Inport
  aIn : Inport  Port=2
  validIn : Inport  Port=3
  validElim : Inport  Port=4
  restart : Inport  Port=5
  Delay{,2..4,6} (5 alike) : Delay  DelayLength=1
  MATLAB Function : MATLAB Function  TreatAsAtomicUnit=on
  xOut : Outport  VectorParamsAs1DForOutWhenUnconnected=off
  yOut : Outport  Port=2  VectorParamsAs1DForOutWhenUnconnected=off
  process : Outport  Port=3  VectorParamsAs1DForOutWhenUnconnected=off
  validOut : Outport  Port=4  VectorParamsAs1DForOutWhenUnconnected=off
  ready : Outport  Port=5  VectorParamsAs1DForOutWhenUnconnected=off
  wires:
  Delay/1 -> MATLAB Function/1(xIn)
  Delay2/1 -> MATLAB Function/2(aIn)
  Delay3/1 -> MATLAB Function/3(validIn)
  Delay4/1 -> MATLAB Function/4(validRowRotationInput)
  Delay6/1 -> MATLAB Function/5(restart)
  xIn/1 -> Delay/1  "A"
  aIn/1 -> Delay2/1
  validIn/1 -> Delay3/1  "validIn"
  validElim/1 -> Delay4/1  "validElim"
  restart/1 -> Delay6/1  "validElim"
  MATLAB Function/1(xOut) -> xOut/1
  MATLAB Function/2(yOut) -> yOut/1
  MATLAB Function/3(processRowRotations) -> process/1
  MATLAB Function/4(validOut) -> validOut/1
  MATLAB Function/5(ready) -> ready/1

== system qless_forgetting_factor_16x16_nofifo/MVDR_QLess_HDL/Complex Partial-Systolic Matrix Solve Using Q-less QR Decomposition with Forgetting Factor Manually Tiled n=16/Complex Partial-Systolic Q-less QR with Forgetting Factor/Complex Partial-Systolic Q-less QR with Forgetting Factor Manually tiled/Complex Partial-Systolic Q-less QR Decomposition with Forgetting Factor Section Constant pivot16/Same Datatype ==
  Data : Inport
  Reference : Inport  Port=2
  Data Type Duplicate : DataTypeDuplicate
  DataOut : Outport  VectorParamsAs1DForOutWhenUnconnected=off
  wires:
  Reference/1 -> Data Type Duplicate/2
  Data/1 -> DataOut/1, Data Type Duplicate/1

== system qless_forgetting_factor_16x16_nofifo/MVDR_QLess_HDL/Complex Partial-Systolic Matrix Solve Using Q-less QR Decomposition with Forgetting Factor Manually Tiled n=16/Complex Partial-Systolic Q-less QR with Forgetting Factor/Complex Partial-Systolic Q-less QR with Forgetting Factor Manually tiled/Complex Partial-Systolic Q-less QR Decomposition with Forgetting Factor Section Constant pivot2/Complex Partial-Systolic Q-less QR Row Rotations ==
  note: The pivot element is already real
  note: Zero-out the imaginary part
      | of the sub-diagonal element
  x : Inport
  y : Inport  Port=2
  validIn : Inport  Port=3
  restart : Inport  Port=4
  Complex Partial-Systolic Q-less QR CORDIC Row Rotation : Subsystem  TreatAsAtomicUnit=on  mask(Real Indexed CORDIC Row Rotation){n=n, pivot=pivot}
      mask prompts: n "fixed:emblib:ColumnsInA"
      mask help: fixed:emblib:RealIdxCORDIC
      mask DialogControl n Prompt: Number of columns in matrix A
  Delay{,1..3,5..8,10,16..18,21} (13 alike) : Delay  DelayLength=1
  Inverse CORDIC Gain1 : Subsystem  mask(Inverse CORDIC Gain){}
      mask help: fixed:emblib:InverseCORDICGainDescription
      mask Display: disp('1/An')
  Inverse CORDIC Gain4 : Subsystem  mask(Inverse CORDIC Gain){}
      mask help: fixed:emblib:InverseCORDICGainDescription
      mask Display: disp('1/An')
  Q-less QR 2nd and 3rd Quadrant Compensation : MATLAB Function  TreatAsAtomicUnit=on
  Q-less QR Rotate First Element To Real1 : Subsystem  TreatAsAtomicUnit=on  mask(Rotate First Element To Real){n=n, pivot=pivot}
      mask prompts: n "fixed:emblib:ColumnsInA"
      mask help: fixed:emblib:RotateFirstElementToRealDescription
      mask DialogControl n Prompt: Number of columns in matrix A
  Set Element To Zero1 : Subsystem  mask(Set Element To Zero){n=n, pivot=pivot}
      mask prompts: n "fixed:emblib:ColumnsInA"
      mask help: fixed:emblib:SetElementToZeroDescription
      mask DialogControl n Prompt: Number of columns in matrix A
  Terminator3 : Terminator
  Unit Delay Enabled Synchronous1 : hdlsllib/Discrete/Unit Delay Enabled Synchronous  InitialCondition=0.0  SampleTime=-1
      settings: SourceProductBaseCode=SL
  Unit Delay Enabled Synchronous3 : hdlsllib/Discrete/Unit Delay Enabled Synchronous  InitialCondition=0.0  SampleTime=-1
      settings: SourceProductBaseCode=SL
  ValidIn to Ready Logic : Subsystem
  ValidIn to Ready Logic1 : Subsystem
  xOut : Outport  VectorParamsAs1DForOutWhenUnconnected=off
  yOut : Outport  Port=2  VectorParamsAs1DForOutWhenUnconnected=off
  validOut : Outport  Port=3  VectorParamsAs1DForOutWhenUnconnected=off
  ready : Outport  Port=4  VectorParamsAs1DForOutWhenUnconnected=off
  wires:
  Delay6/1 -> xOut/1
  Complex Partial-Systolic Q-less QR CORDIC Row Rotation/1(xOut) -> Delay17/1
  Q-less QR 2nd and 3rd Quadrant Compensation/1(xOut) -> Delay/1
  Q-less QR 2nd and 3rd Quadrant Compensation/2(yOut) -> Delay1/1
  Delay/1 -> Complex Partial-Systolic Q-less QR CORDIC Row Rotation/1(x)
  Q-less QR Rotate First Element To Real1/2(validOut) -> Unit Delay Enabled Synchronous3/2, Delay16/1
  Q-less QR Rotate First Element To Real1/1(xOut) -> Delay2/1
  Delay1/1 -> Complex Partial-Systolic Q-less QR CORDIC Row Rotation/2(y)
  restart/1 -> Q-less QR Rotate First Element To Real1/3(restart), Complex Partial-Systolic Q-less QR CORDIC Row Rotation/4(restart)
  Delay5/1 -> ValidIn to Ready Logic/2(validIn), Complex Partial-Systolic Q-less QR CORDIC Row Rotation/3(validIn)
  Complex Partial-Systolic Q-less QR CORDIC Row Rotation/4(ready) -> ValidIn to Ready Logic/1(readyIn)
  Complex Partial-Systolic Q-less QR CORDIC Row Rotation/3(validOut) -> Delay21/1
  Complex Partial-Systolic Q-less QR CORDIC Row Rotation/2(yOut) -> Delay18/1
  y/1 -> Delay3/1
  Delay10/1 -> validOut/1
  ValidIn to Ready Logic/1(readyOut) -> ValidIn to Ready Logic1/1(readyIn)
  Delay7/1 -> Set Element To Zero1/1(u)
  Q-less QR Rotate First Element To Real1/3(ready) -> Terminator3/1
  ValidIn to Ready Logic1/1(readyOut) -> ready/1
  Delay21/1 -> Delay10/1
  Delay18/1 -> Inverse CORDIC Gain1/1(u)
  Delay17/1 -> Inverse CORDIC Gain4/1(u)
  Inverse CORDIC Gain4/1(y) -> Delay6/1
  Inverse CORDIC Gain1/1(y) -> Delay7/1
  validIn/1 -> Unit Delay Enabled Synchronous1/2, Delay8/1
  Delay16/1 -> ValidIn to Ready Logic1/2(validIn), Delay5/1
  Delay2/1 -> Q-less QR 2nd and 3rd Quadrant Compensation/2(y)
  Unit Delay Enabled Synchronous3/1 -> Q-less QR 2nd and 3rd Quadrant Compensation/1(x)
  Unit Delay Enabled Synchronous1/1 -> Unit Delay Enabled Synchronous3/1
  x/1 -> Unit Delay Enabled Synchronous1/1
  Delay3/1 -> Q-less QR Rotate First Element To Real1/1(x)
  Delay8/1 -> Q-less QR Rotate First Element To Real1/2(validIn)
  Set Element To Zero1/1(y) -> yOut/1

== system qless_forgetting_factor_16x16_nofifo/MVDR_QLess_HDL/Complex Partial-Systolic Matrix Solve Using Q-less QR Decomposition with Forgetting Factor Manually Tiled n=16/Complex Partial-Systolic Q-less QR with Forgetting Factor/Complex Partial-Systolic Q-less QR with Forgetting Factor Manually tiled/Complex Partial-Systolic Q-less QR Decomposition with Forgetting Factor Section Constant pivot2/Partial-Systolic Q-less QR with Forgetting Factor Memory Controller ==
  xIn : Inport
  aIn : Inport  Port=2
  validIn : Inport  Port=3
  validElim : Inport  Port=4
  restart : Inport  Port=5
  Delay{,2..4,6} (5 alike) : Delay  DelayLength=1
  MATLAB Function : MATLAB Function  TreatAsAtomicUnit=on
  xOut : Outport  VectorParamsAs1DForOutWhenUnconnected=off
  yOut : Outport  Port=2  VectorParamsAs1DForOutWhenUnconnected=off
  process : Outport  Port=3  VectorParamsAs1DForOutWhenUnconnected=off
  validOut : Outport  Port=4  VectorParamsAs1DForOutWhenUnconnected=off
  ready : Outport  Port=5  VectorParamsAs1DForOutWhenUnconnected=off
  wires:
  Delay/1 -> MATLAB Function/1(xIn)
  Delay2/1 -> MATLAB Function/2(aIn)
  Delay3/1 -> MATLAB Function/3(validIn)
  Delay4/1 -> MATLAB Function/4(validRowRotationInput)
  Delay6/1 -> MATLAB Function/5(restart)
  xIn/1 -> Delay/1  "A"
  aIn/1 -> Delay2/1
  validIn/1 -> Delay3/1  "validIn"
  validElim/1 -> Delay4/1  "validElim"
  restart/1 -> Delay6/1  "validElim"
  MATLAB Function/1(xOut) -> xOut/1
  MATLAB Function/2(yOut) -> yOut/1
  MATLAB Function/3(processRowRotations) -> process/1
  MATLAB Function/4(validOut) -> validOut/1
  MATLAB Function/5(ready) -> ready/1

== system qless_forgetting_factor_16x16_nofifo/MVDR_QLess_HDL/Complex Partial-Systolic Matrix Solve Using Q-less QR Decomposition with Forgetting Factor Manually Tiled n=16/Complex Partial-Systolic Q-less QR with Forgetting Factor/Complex Partial-Systolic Q-less QR with Forgetting Factor Manually tiled/Complex Partial-Systolic Q-less QR Decomposition with Forgetting Factor Section Constant pivot2/Same Datatype ==
  Data : Inport
  Reference : Inport  Port=2
  Data Type Duplicate : DataTypeDuplicate
  DataOut : Outport  VectorParamsAs1DForOutWhenUnconnected=off
  wires:
  Reference/1 -> Data Type Duplicate/2
  Data/1 -> DataOut/1, Data Type Duplicate/1

== system qless_forgetting_factor_16x16_nofifo/MVDR_QLess_HDL/Complex Partial-Systolic Matrix Solve Using Q-less QR Decomposition with Forgetting Factor Manually Tiled n=16/Complex Partial-Systolic Q-less QR with Forgetting Factor/Complex Partial-Systolic Q-less QR with Forgetting Factor Manually tiled/Complex Partial-Systolic Q-less QR Decomposition with Forgetting Factor Section Constant pivot3/Complex Partial-Systolic Q-less QR Row Rotations ==
  note: The pivot element is already real
  note: Zero-out the imaginary part
      | of the sub-diagonal element
  x : Inport
  y : Inport  Port=2
  validIn : Inport  Port=3
  restart : Inport  Port=4
  Complex Partial-Systolic Q-less QR CORDIC Row Rotation : Subsystem  TreatAsAtomicUnit=on  mask(Real Indexed CORDIC Row Rotation){n=n, pivot=pivot}
      mask prompts: n "fixed:emblib:ColumnsInA"
      mask help: fixed:emblib:RealIdxCORDIC
      mask DialogControl n Prompt: Number of columns in matrix A
  Delay{,1..3,5..8,10,16..18,21} (13 alike) : Delay  DelayLength=1
  Inverse CORDIC Gain1 : Subsystem  mask(Inverse CORDIC Gain){}
      mask help: fixed:emblib:InverseCORDICGainDescription
      mask Display: disp('1/An')
  Inverse CORDIC Gain4 : Subsystem  mask(Inverse CORDIC Gain){}
      mask help: fixed:emblib:InverseCORDICGainDescription
      mask Display: disp('1/An')
  Q-less QR 2nd and 3rd Quadrant Compensation : MATLAB Function  TreatAsAtomicUnit=on
  Q-less QR Rotate First Element To Real1 : Subsystem  TreatAsAtomicUnit=on  mask(Rotate First Element To Real){n=n, pivot=pivot}
      mask prompts: n "fixed:emblib:ColumnsInA"
      mask help: fixed:emblib:RotateFirstElementToRealDescription
      mask DialogControl n Prompt: Number of columns in matrix A
  Set Element To Zero1 : Subsystem  mask(Set Element To Zero){n=n, pivot=pivot}
      mask prompts: n "fixed:emblib:ColumnsInA"
      mask help: fixed:emblib:SetElementToZeroDescription
      mask DialogControl n Prompt: Number of columns in matrix A
  Terminator3 : Terminator
  Unit Delay Enabled Synchronous1 : hdlsllib/Discrete/Unit Delay Enabled Synchronous  InitialCondition=0.0  SampleTime=-1
      settings: SourceProductBaseCode=SL
  Unit Delay Enabled Synchronous3 : hdlsllib/Discrete/Unit Delay Enabled Synchronous  InitialCondition=0.0  SampleTime=-1
      settings: SourceProductBaseCode=SL
  ValidIn to Ready Logic : Subsystem
  ValidIn to Ready Logic1 : Subsystem
  xOut : Outport  VectorParamsAs1DForOutWhenUnconnected=off
  yOut : Outport  Port=2  VectorParamsAs1DForOutWhenUnconnected=off
  validOut : Outport  Port=3  VectorParamsAs1DForOutWhenUnconnected=off
  ready : Outport  Port=4  VectorParamsAs1DForOutWhenUnconnected=off
  wires:
  Delay6/1 -> xOut/1
  Complex Partial-Systolic Q-less QR CORDIC Row Rotation/1(xOut) -> Delay17/1
  Q-less QR 2nd and 3rd Quadrant Compensation/1(xOut) -> Delay/1
  Q-less QR 2nd and 3rd Quadrant Compensation/2(yOut) -> Delay1/1
  Delay/1 -> Complex Partial-Systolic Q-less QR CORDIC Row Rotation/1(x)
  Q-less QR Rotate First Element To Real1/2(validOut) -> Unit Delay Enabled Synchronous3/2, Delay16/1
  Q-less QR Rotate First Element To Real1/1(xOut) -> Delay2/1
  Delay1/1 -> Complex Partial-Systolic Q-less QR CORDIC Row Rotation/2(y)
  restart/1 -> Q-less QR Rotate First Element To Real1/3(restart), Complex Partial-Systolic Q-less QR CORDIC Row Rotation/4(restart)
  Delay5/1 -> ValidIn to Ready Logic/2(validIn), Complex Partial-Systolic Q-less QR CORDIC Row Rotation/3(validIn)
  Complex Partial-Systolic Q-less QR CORDIC Row Rotation/4(ready) -> ValidIn to Ready Logic/1(readyIn)
  Complex Partial-Systolic Q-less QR CORDIC Row Rotation/3(validOut) -> Delay21/1
  Complex Partial-Systolic Q-less QR CORDIC Row Rotation/2(yOut) -> Delay18/1
  y/1 -> Delay3/1
  Delay10/1 -> validOut/1
  ValidIn to Ready Logic/1(readyOut) -> ValidIn to Ready Logic1/1(readyIn)
  Delay7/1 -> Set Element To Zero1/1(u)
  Q-less QR Rotate First Element To Real1/3(ready) -> Terminator3/1
  ValidIn to Ready Logic1/1(readyOut) -> ready/1
  Delay21/1 -> Delay10/1
  Delay18/1 -> Inverse CORDIC Gain1/1(u)
  Delay17/1 -> Inverse CORDIC Gain4/1(u)
  Inverse CORDIC Gain4/1(y) -> Delay6/1
  Inverse CORDIC Gain1/1(y) -> Delay7/1
  validIn/1 -> Unit Delay Enabled Synchronous1/2, Delay8/1
  Delay16/1 -> ValidIn to Ready Logic1/2(validIn), Delay5/1
  Delay2/1 -> Q-less QR 2nd and 3rd Quadrant Compensation/2(y)
  Unit Delay Enabled Synchronous3/1 -> Q-less QR 2nd and 3rd Quadrant Compensation/1(x)
  Unit Delay Enabled Synchronous1/1 -> Unit Delay Enabled Synchronous3/1
  x/1 -> Unit Delay Enabled Synchronous1/1
  Delay3/1 -> Q-less QR Rotate First Element To Real1/1(x)
  Delay8/1 -> Q-less QR Rotate First Element To Real1/2(validIn)
  Set Element To Zero1/1(y) -> yOut/1
